simulink subsystem "REG32BLOCK_SS"  (R2022a)
settings: Solver=VariableStepAuto  StartTime=0.0  StopTime=10.0  RelTol=1e-3
libraries: hdlBasic x6
settings Model: Creator=viktor  LastModifiedBy=viktor

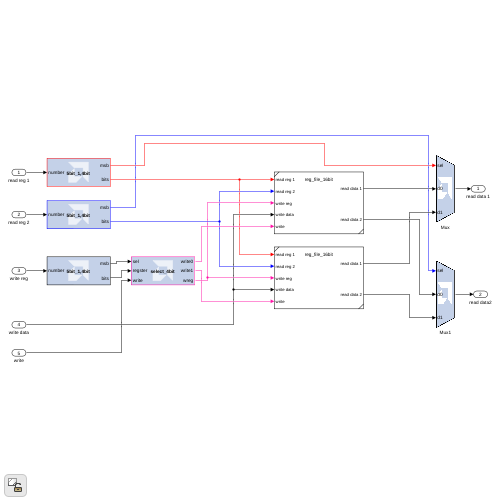
[thumbnail: Simulink's stored preview of the top-level diagram]
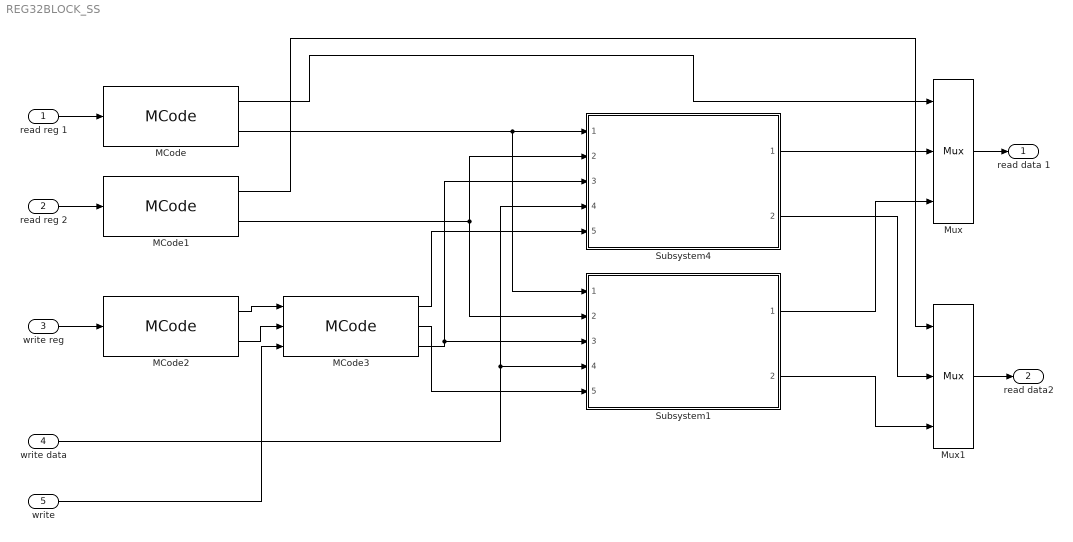
== system REG32BLOCK_SS ==
  read reg 1 : Inport
  read reg 2 : Inport  Port=2
  write reg : Inport  Port=3
  write data : Inport  Port=4
  write : Inport  Port=5
  MCode : hdlBasic/MCode  mfname=5bit_1,4bit  explicit_period=off  period=1  iptable={ 'number', '' }  optable={ 'msb', 'off'; 'bits', 'off' }  enable_stdout=off  enable_debug=off  suppress_output='on'  defparams={}  hide_port_list={}  block_type=mcode  block_width=444  block_height=788
      settings: infoedit=Pass input values to a MATLAB function for evaluation in Xilinx fixed-point type. The input ports of the block are input arguments of the function. The output ports of the block are output arguments of the function.
  MCode1 : hdlBasic/MCode  mfname=5bit_1,4bit  explicit_period=off  period=1  iptable={ 'number', '' }  optable={ 'msb', 'off'; 'bits', 'off' }  enable_stdout=off  enable_debug=off  suppress_output='on'  defparams={}  hide_port_list={}  block_type=mcode  block_width=444  block_height=788
      settings: infoedit=Pass input values to a MATLAB function for evaluation in Xilinx fixed-point type. The input ports of the block are input arguments of the function. The output ports of the block are output arguments of the function.
  MCode2 : hdlBasic/MCode  mfname=5bit_1,4bit  explicit_period=off  period=1  iptable={ 'number', '' }  optable={ 'msb', 'off'; 'bits', 'off' }  enable_stdout=off  enable_debug=off  suppress_output='on'  defparams={}  hide_port_list={}  block_type=mcode  block_width=444  block_height=788
      settings: infoedit=Pass input values to a MATLAB function for evaluation in Xilinx fixed-point type. The input ports of the block are input arguments of the function. The output ports of the block are output arguments of the function.
  MCode3 : hdlBasic/MCode  mfname=select_4bit  explicit_period=off  period=1  iptable={ 'sel', ''; 'reg', ''; 'write', '' }  optable={ 'write0', 'off'; 'write1', 'off'; 'wreg', 'off' }  enable_stdout=off  enable_debug=off  suppress_output='on'  defparams={}  hide_port_list={}  block_type=mcode  block_width=444  block_height=788
      settings: infoedit=Pass input values to a MATLAB function for evaluation in Xilinx fixed-point type. The input ports of the block are input arguments of the function. The output ports of the block are output arguments of the function.
  Mux : hdlBasic/Mux  inputs=2  en=off  latency=0  precision=Full  arith_type=Unsigned  n_bits=16  bin_pt=14  quantization=Truncate  overflow=Wrap  XmcBlockStatus=1  maskContainerNames=tabcontainer1  block_type=mux  block_config=sysgen:Mux_config
  Mux1 : hdlBasic/Mux  inputs=2  en=off  latency=0  precision=Full  arith_type=Unsigned  n_bits=16  bin_pt=14  quantization=Truncate  overflow=Wrap  XmcBlockStatus=1  maskContainerNames=tabcontainer1  block_type=mux  block_config=sysgen:Mux_config
  Subsystem1 : Subsystem  ReferencedSubsystem=reg_file_16bit
  Subsystem4 : Subsystem  ReferencedSubsystem=reg_file_16bit
  read data 1 : Outport
  read data2 : Outport  Port=2
  wires:
  MCode2/1 -> MCode3/1
  Subsystem4/2 -> Mux1/2
  Subsystem4/1 -> Mux/2
  MCode2/2 -> MCode3/2
  MCode/1 -> Mux/1
  MCode3/2 -> Subsystem1/5
  write/1 -> MCode3/3
  write reg/1 -> MCode2/1
  Mux1/1 -> read data2/1
  read reg 2/1 -> MCode1/1
  MCode3/3 -> Subsystem4/3, Subsystem1/3
  read reg 1/1 -> MCode/1
  MCode1/2 -> Subsystem4/2, Subsystem1/2
  Mux/1 -> read data 1/1
  write data/1 -> Subsystem1/4, Subsystem4/4
  MCode3/1 -> Subsystem4/5
  MCode1/1 -> Mux1/1
  Subsystem1/2 -> Mux1/3
  Subsystem1/1 -> Mux/3
  MCode/2 -> Subsystem4/1, Subsystem1/1
